simulink model "Datos1R16"  (R2022b)
settings: Solver=VariableStepAuto  StartTime=0.0  StopTime=10.0  RelTol=1e-3
libraries: simulink x1
settings Model: Creator=PC-LUISMIGUEL  LastModifiedBy=PC-LUISMIGUEL

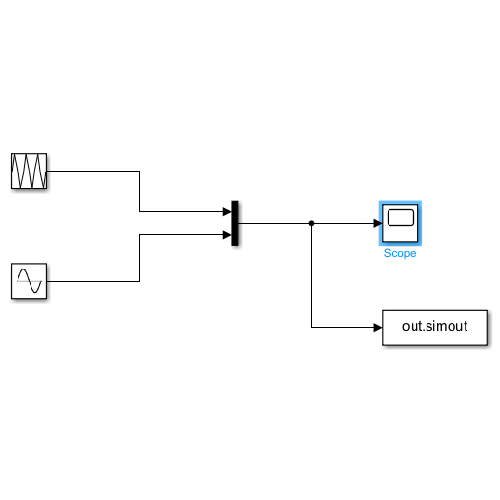
[thumbnail: Simulink's stored preview of the top-level diagram]
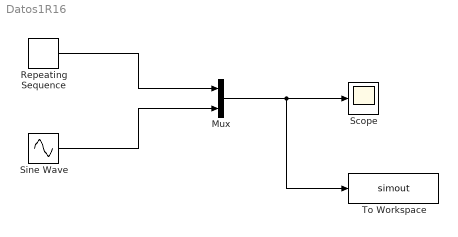
== system Datos1R16 ==
  Mux : Mux  Inputs=2
  Repeating Sequence : simulink/Sources/Repeating Sequence  rep_seq_t=[0 1 2 3 4]  rep_seq_y=[0 1 0 -1 0]
  Scope : Scope
  Sine Wave : Sin  Frequency=2*pi/4  SampleTime=0
  To Workspace : ToWorkspace  VariableName=simout  SaveFormat=Timeseries  SampleTime=-1
  wires:
  Sine Wave/1 -> Mux/2
  Mux/1 -> Scope/1, To Workspace/1
  Repeating Sequence/1 -> Mux/1
